simulink model "static_split_junction_test"  (R2014b)
settings: Solver=ode45  StartTime=0.0  StopTime=10.0  RelTol=1e-3
libraries: DAEMOT_Lib x7
settings Model: Creator=pangbor2  LastModifiedBy=pangbor2

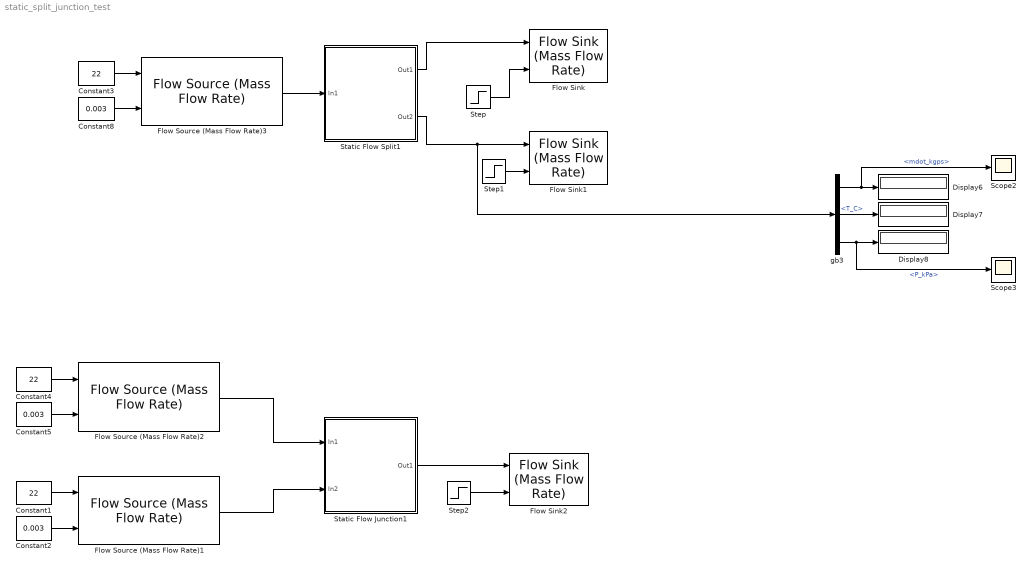
== system static_split_junction_test ==
  Constant1 : Constant  Value=22
  Constant2 : Constant  Value=0.003
  Constant3 : Constant  Value=22
  Constant4 : Constant  Value=22
  Constant5 : Constant  Value=0.003
  Constant8 : Constant  Value=0.003
  Display6 : Display
  Display7 : Display
  Display8 : Display
  Flow Sink : DAEMOT_Lib/Components/Flow Sink (Mass Flow Rate)  M_ext=on  M=0  T_ext=on  T=0  P_ext=on  P=0
  Flow Sink1 : DAEMOT_Lib/Components/Flow Sink (Mass Flow Rate)  M_ext=on  M=0  T_ext=on  T=0  P_ext=on  P=0
  Flow Sink2 : DAEMOT_Lib/Components/Flow Sink (Mass Flow Rate)  M_ext=on  M=0  T_ext=on  T=0  P_ext=on  P=0
  Flow Source (Mass Flow Rate)1 : DAEMOT_Lib/Components/Flow Source (Mass Flow Rate)  M_ext=on  M=0  T_ext=on  T=0  P_ext=on  P=0
  Flow Source (Mass Flow Rate)2 : DAEMOT_Lib/Components/Flow Source (Mass Flow Rate)  M_ext=on  M=0  T_ext=on  T=0  P_ext=on  P=0
  Flow Source (Mass Flow Rate)3 : DAEMOT_Lib/Components/Flow Source (Mass Flow Rate)  M_ext=on  M=0  T_ext=on  T=0  P_ext=on  P=0
  Scope2 : Scope
      settings: SaveName=ScopeData2
  Scope3 : Scope
      settings: SaveName=ScopeData3
  Static Flow Junction1 : Subsystem  AncestorBlock=DAEMOT_Lib/Components/Static Flow Junction  mask(Static Flow Junction){Num_In=2}
      mask prompts: Num_In "Number of Inlet Flows"
      mask help: Joins multiple flows into a single exit flow. Mass flow rates are taken from the upstream blocks. Note that the library link of the block is disabled when it is imported into a model.
      mask init:
      | h      = get_param(gcb,'handle');   % Get block handle
      | blk    = gcb; 
      | hblock = get(h);     % Parse out handles structure 
      | 
      | % delete any previous inports and bus selectors
      | for i = str2num(hblock.Num_In)+1:hblock.Ports(1)
      |     delete_block([blk,'/In',num2str(i)])
      |     delete_block([blk,'/b',num2str(i)])
      |     delete_block([blk,'/gm',num2str(i)])
      |     delete_block([blk,'/gt',num2str(i)])
      |     delete_block([blk,'/gp',num2str(i)])
      |     delete_block([blk,'/m',num2str(i)])
      |     delete_block([blk,'/p',num2str(i)])
      |     delete_block([blk,'/m2_',num2str(i)])
      |     delete_block([blk,'/t2_',num2str(i)])
      |     delete_block([blk,'/Divide',num2str(i)])
      |     
      | 	delete_unconnected_lines(blk)
      | end
      | 
      | % add the correct number of inputs to the add blocks
      | set_param([blk,'/Add'],'Inputs',char(repmat('+',1,str2num(hblock.Num_In))))
      | set_param([blk,'/Add1'],'Inputs',char(repmat('+',1,str2num(hblock.Num_In))))
      | set_param([blk,'/Add2'],'Inputs',char(repmat('+',1,str2num(hblock.Num_In))))
      | set_param([blk,'/Constant'],'Value',char(hblock.Num_In))
      | 
      | % generate inports, bus selectors, and route lines to each vector concat
      | for i = hblock.Ports(1)+1:str2num(hblock.Num_In)
      |     
      |     % add blocks
      |     add_block('simulink/Ports & Subsystems/In1',     [blk,'/In',num2str(i)],    'Position',[120 i*80-7 150 i*80+7]);         % adding inport   
      |     add_block([blk,'/b1'],                           [blk,'/b',num2str(i)],     'Position',[200 i*80-20+20-18 205 i*80-2+20+2]);         % adding inport
      |     add_block('simulink/Signal Routing/Goto',        [blk,'/gm',num2str(i)],    'Position',[260 i*80-17 340 i*80-3]);         % adding inport
      |     add_block('simulink/Signal Routing/Goto',        [blk,'/gt',num2str(i)],    'Position',[260 i*80+3 340 i*80+17]);         % adding inport
      |     add_block('simulink/Signal Routing/Goto',        [blk,'/gp',num2str(i)],    'Position',[260 i*80+6 340 i*80+20]);         % adding inport
      |     add_block('simulink/Signal Routing/From',        [blk,'/m',num2str(i)],     'Position',[410 i*80-20 490 i*80-2]);         % adding inport
      |     add_block('simulink/Signal Routing/From',        [blk,'/p',num2str(i)],     'Position',[1445 i*80-20 1525 i*80-2]);         % adding inport
      |     add_block('simulink/Signal Routing/From',        [blk,'/m2_',num2str(i)],   'Position',[730 i*80-20 810 i*80-2]);         % adding inport
      |     add_block('simulink/Signal Routing/From',        [blk,'/t2_',num2str(i)],   'Position',[730 i*80-20+24 810 i*80+24]);         % adding inport
      |     add_block([blk,'/Divide1'],                      [blk,'/Divide',num2str(i)],'Position',[825 i*80-20-7 841 i*80+27]);         % adding inport
      |     
      |     % set goto and from tags
      |     set_param([blk,'/gm',num2str(i)],'GotoTag',char(horzcat('m_in',num2str(i))))
      |     set_param([blk,'/gt',num2str(i)],'GotoTag',char(horzcat('T_in',num2str(i))))
      |     set_param([blk,'/gp',num2str(i)],'GotoTag',char(horzcat('P_in',num2str(i))))
      |     set_param([blk,'/m',num2str(i)],'GotoTag',char(horzcat('m_in',num2str(i))))
      |     set_param([blk,'/p',num2str(i)],'GotoTag',char(horzcat('P_in',num2str(i))))
      |     set_param([blk,'/m2_',num2str(i)],'GotoTag',char(horzcat('m_in',num2str(i))))
      |     set_param([blk,'/t2_',num2str(i)],'GotoTag',char(horzcat('T_in',num2str(i))))
      |    % set_param([blk,'/b',num2str(i)],'Outputs','3')
      |     
      |     % add lines
      |     add_line(blk,['In',num2str(i),'/1'], ['b',num2str(i),'/1'],'AutoRouting','on')
      |     add_line(blk,['b',num2str(i),'/1'],  ['gm',num2str(i),'/1'],'AutoRouting','on')
      |     add_line(blk,['b',num2str(i),'/2'],  ['gt',num2str(i),'/1'],'AutoRouting','on')
      |     add_line(blk,['b',num2str(i),'/3'],  ['gp',num2str(i),'/1'],'AutoRouting','on')
      |     add_line(blk,['m',num2str(i),'/1'],  ['Add/',num2str(i)],'AutoRouting','on')
      |     add_line(blk,['p',num2str(i),'/1'],  ['Add2/',num2str(i)],'AutoRouting','on')
      |     add_line(blk,['m2_',num2str(i),'/1'], ['Divide',num2str(i),'/1'],'AutoRouting','on')
      |     add_line(blk,['t2_',num2str(i),'/1'], ['Divide',num2str(i),'/2'],'AutoRouting','on')
      |     add_line(blk,['Divide',num2str(i),'/1'], ['Add1/',num2str(i)],'AutoRouting','on')
      |     
      |     % set goto and from background colors
      |     set_param([blk,'/gm',num2str(i)],'BackgroundColor','yellow') 
      |     set_param([blk,'/gt',num2str(i)],'BackgroundColor','yellow') 
      |     set_param([blk,'/gp',num2str(i)],'BackgroundColor','yellow') 
      |     set_param([blk,'/m',num2str(i)],'BackgroundColor','cyan') 
      |     set_param([blk,'/p',num2str(i)],'BackgroundColor','cyan') 
      |     set_param([blk,'/m2_',num2str(i)],'BackgroundColor','cyan') 
      |     set_param([blk,'/t2_',num2str(i)],'BackgroundColor','cyan') 
      |         
      | end
      settings: CopyFcn=|
      | h      = get_param(gcb,'handle');   % Get block handle
      | blk    = gcb;
      | 
      | set_param(blk, 'LinkStatus', 'inactive')
      mask Display:
      | image(fliplr(imread('Split.jpg')));
      | 
      | text(0.5,0.95,['{\bf Static Flow Junction}'],'TexMode','on','horizontalAlignment', 'center')
      | 
      | port_label('output',1,['Flow Out'])
      | 
      | h      = get_param(gcb,'handle');   % Get block handle
      | blk    = gcb;
      | hblock = get(h);     % Parse out handles structure
      | for i = 1:str2num(hblock.Num_In)
      |     port_label('input',i,horzcat('Flow In #',num2str(i)))
      | end
  Static Flow Split1 : Subsystem  AncestorBlock=DAEMOT_Lib/Components/Static Flow Split  mask(Static Flow Split){Num_Out=2}
      mask prompts: Num_Out "Number of Outlet Flows"
      mask help: Splits an inlet flow into multiple exit flows. Mass flow rates are taken from the downstream blocks. Note that the library link of the block is disabled when it is imported into a model.
      mask init:
      | h      = get_param(gcb,'handle');   % Get block handle
      | blk    = gcb; 
      | hblock = get(h);     % Parse out handles structure 
      | 
      | % delete any previous inports and bus selectors
      | for i = str2num(hblock.Num_Out)+1:hblock.Ports(2)
      |    delete_block([blk,'/Out',num2str(i)])
      |    delete_block([blk,'/m',num2str(i)])
      |    delete_block([blk,'/t',num2str(i)])
      |    delete_block([blk,'/p',num2str(i)])
      |    delete_block([blk,'/b',num2str(i)])
      |    delete_block([blk,'/Source',num2str(i)])
      |    delete_block([blk,'/g',num2str(i)])
      |    
      |    delete_unconnected_lines(blk)
      | end
      | 
      | % add the correct number of inputs to the add block
      | set_param([blk,'/Add'],'Inputs',char(repmat('+',1,str2num(hblock.Num_Out))))
      | 
      | % generate inports, bus selectors, and route lines to each vector concat
      | for i = hblock.Ports(2)+1:str2num(hblock.Num_Out)
      |     
      |     % add blocks
      |     add_block('simulink/Ports & Subsystems/Out1',   [blk,'/Out',num2str(i)],   'Position',[30 i*80-25+20 60 i*80-12+20]);         % adding inport
      |     add_block('simulink/Signal Routing/From',       [blk,'/m',num2str(i)],     'Position',[-150 i*80-20 -70 i*80-2]);         % adding inport
      |     add_block('simulink/Signal Routing/From',       [blk,'/t',num2str(i)],     'Position',[-150 i*80-20+20 -70 i*80-2+20]);         % adding inport
      |     add_block('simulink/Signal Routing/From',       [blk,'/p',num2str(i)],     'Position',[-150 i*80-20+40 -70 i*80-2+40]);         % adding inport
      |     add_block('simulink/Signal Routing/Bus Creator',[blk,'/b',num2str(i)],     'Position',[5 i*80-20+20-18 10 i*80-2+20+2]);         % adding inport
      |     add_block('DAEMOT_Lib/Support Functions/Source',[blk,'/Source',num2str(i)],'Position',[395 i*80-14 460 i*80+14]);         % adding inport
      |     add_block('simulink/Signal Routing/Goto',       [blk,'/g',num2str(i)],     'Position',[505 i*80-9 585 i*80+9]);         % adding inport
      |     
      |     % set goto and from tags
      |     set_param([blk,'/m',num2str(i)],'GotoTag',char(horzcat('m_dot',num2str(i))))
      |     set_param([blk,'/t',num2str(i)],'GotoTag',char('T_in'))
      |     set_param([blk,'/p',num2str(i)],'GotoTag',char('P_in'))
      |     set_param([blk,'/g',num2str(i)],'GotoTag',char(['m_dot',num2str(i)]))
      |     set_param([blk,'/b',num2str(i)],'Inputs','3')
      |     
      |     % set goto and from background colors
      |     set_param([blk,'/t',num2str(i)],'BackgroundColor','cyan')
      |     set_param([blk,'/m',num2str(i)],'BackgroundColor','cyan') 
      |     set_param([blk,'/p',num2str(i)],'BackgroundColor','cyan') 
      |     set_param([blk,'/g',num2str(i)],'BackgroundColor','yellow')    
      |     
      |     % add lines
      |     add_line(blk,['m',num2str(i),'/1'],['b',num2str(i),'/1'],'AutoRouting','on')
      |     add_line(blk,['t',num2str(i),'/1'],['b',num2str(i),'/2'],'AutoRouting','on')
      |     add_line(blk,['p',num2str(i),'/1'],['b',num2str(i),'/3'],'AutoRouting','on')
      |     add_line(blk,['b',num2str(i),'/1'],['Out',num2str(i),'/1'],'AutoRouting','on')
      |     add_line(blk,['Source',num2str(i),'/1'],['g',num2str(i),'/1'],'AutoRouting','on')
      |     add_line(blk,['Source',num2str(i),'/1'],['Add/',num2str(i)],'AutoRouting','on')
      |     
      |     % set line names for mass flow bus
      |     p = get_param([blk,'/m',num2str(i)], 'PortHandles');
      |     l = get_param(p.Outport,'Line');
      |     set_param(l,'Name','mdot_kgps')
      |     
      |     % set line names for temperature bus
      |     p = get_param([blk,'/t',num2str(i)], 'PortHandles');
      |     l = get_param(p.Outport,'Line');
      |     set_param(l,'Name','T_C')
      |     
      |     % set line names for pressure bus
      |     p = get_param([blk,'/p',num2str(i)], 'PortHandles');
      |     l = get_param(p.Outport,'Line');
      |     set_param(l,'Name','P_kPa')
      | end
      | 
      | clear h blk hblock
      settings: CopyFcn=|
      | h      = get_param(gcb,'handle');   % Get block handle
      | blk    = gcb;
      | 
      | set_param(blk, 'LinkStatus', 'inactive')
      mask Display:
      | image(imread('Split.jpg'));
      | 
      | text(0.5,0.95,['{\bf Static Flow Split}'],'TexMode','on','horizontalAlignment', 'center')
      | 
      | port_label('input',1,['Flow In'])
      | 
      | h      = get_param(gcb,'handle');   % Get block handle
      | blk    = gcb;
      | hblock = get(h);     % Parse out handles structure
      | for i = 1:str2num(hblock.Num_Out)
      |     port_label('output',i,horzcat('Flow Out #',num2str(i)))
      | end
  Step : Step  Time=100  Before=.002  After=.003  SampleTime=0
  Step1 : Step  Time=100  Before=.002  After=.003  SampleTime=0
  Step2 : Step  Time=100  Before=.002  After=.003  SampleTime=0
  gb3 : BusSelector  OutputSignals=mdot_kgps,T_C,P_kPa
  wires:
  Flow Source (Mass Flow Rate)3/1 -> Static Flow Split1/1(In1)
  Step/1 -> Flow Sink/2
  Static Flow Split1/1(Out1) -> Flow Sink/1
  Step1/1 -> Flow Sink1/2
  Step2/1 -> Flow Sink2/2
  Static Flow Junction1/1(Out1) -> Flow Sink2/1
  gb3/2 -> Display7/1  "<T_C>"
  gb3/1 -> Scope2/1, Display6/1  "<mdot_kgps>"
  Static Flow Split1/2(Out2) -> gb3/1, Flow Sink1/1
  gb3/3 -> Scope3/1, Display8/1  "<P_kPa>"
  Constant8/1 -> Flow Source (Mass Flow Rate)3/2
  Constant3/1 -> Flow Source (Mass Flow Rate)3/1
  Constant5/1 -> Flow Source (Mass Flow Rate)2/2
  Constant4/1 -> Flow Source (Mass Flow Rate)2/1
  Constant2/1 -> Flow Source (Mass Flow Rate)1/2
  Constant1/1 -> Flow Source (Mass Flow Rate)1/1
  Flow Source (Mass Flow Rate)2/1 -> Static Flow Junction1/1(In1)
  Flow Source (Mass Flow Rate)1/1 -> Static Flow Junction1/2(In2)

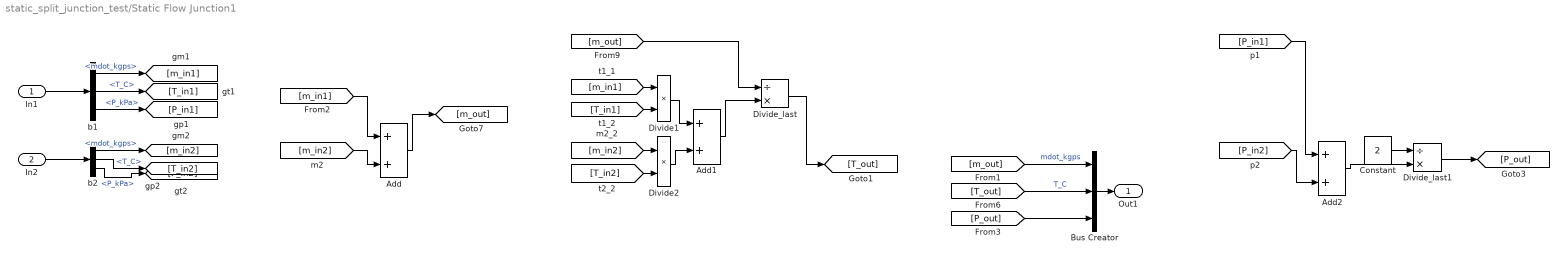
== system static_split_junction_test/Static Flow Junction1 ==
  In1 : Inport
  In2 : Inport  Port=2
  Add : Sum
  Add1 : Sum
  Add2 : Sum
  Bus Creator : BusCreator  Inputs=3
  Constant : Constant  Value=2
  Divide1 : Product  Inputs=**
  Divide2 : Product  Inputs=**
  Divide_last : Product  Inputs=/*
  Divide_last1 : Product  Inputs=/*
  b1 : BusSelector  OutputSignals=mdot_kgps,T_C,P_kPa
  b2 : BusSelector  OutputSignals=mdot_kgps,T_C,P_kPa
  Out1 : Outport
  wires:
  Divide1/1 -> Add1/1
  Add1/1 -> Divide_last/2
  [T_in1] -> Divide1/2
  [m_in1] -> Divide1/1
  Divide_last/1 -> [T_out]
  [m_in1] -> Add/1
  Add/1 -> [m_out]
  [T_out] -> Bus Creator/2  "T_C"
  [m_out] -> Bus Creator/1  "mdot_kgps"
  Bus Creator/1 -> Out1/1
  [m_out] -> Divide_last/1
  [P_out] -> Bus Creator/3
  b1/1 -> [m_in1]  "<mdot_kgps>"
  b1/2 -> [T_in1]  "<T_C>"
  In1/1 -> b1/1
  b1/3 -> [P_in1]  "<P_kPa>"
  [P_in1] -> Add2/1
  Add2/1 -> Divide_last1/2
  Divide_last1/1 -> [P_out]
  Constant/1 -> Divide_last1/1
  In2/1 -> b2/1
  b2/1 -> [m_in2]  "<mdot_kgps>"
  b2/2 -> [T_in2]  "<T_C>"
  b2/3 -> [P_in2]  "<P_kPa>"
  [m_in2] -> Add/2
  [P_in2] -> Add2/2
  [m_in2] -> Divide2/1
  [T_in2] -> Divide2/2
  Divide2/1 -> Add1/2

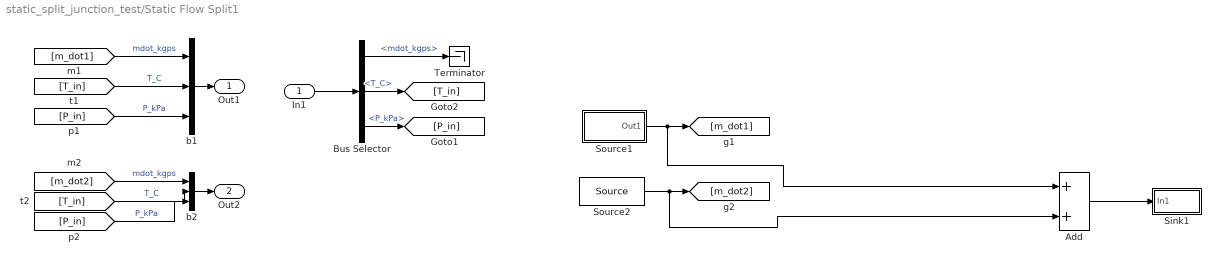
== system static_split_junction_test/Static Flow Split1 ==
  In1 : Inport
  Add : Sum
  Bus Selector : BusSelector  OutputSignals=mdot_kgps,T_C,P_kPa
  Sink1 : Subsystem
      settings: CopyFcn=rev_comms_sink()  NameChangeFcn=rev_comms_sink()
      mask Display: text(0.25,0.5,'Sink')
  Source1 : Subsystem
      mask init:
      | n_src = gcb;
      | n_src = str2num(n_src(end));
      | 
      | rev_comms_source(n_src);
      mask Display: text(0.25,0.5,'Source')
  Source2 : DAEMOT_Lib/Support Functions/Source
  Terminator : Terminator
  b1 : BusCreator  Inputs=3
  b2 : BusCreator  Inputs=3
  Out1 : Outport
  Out2 : Outport  Port=2
  wires:
  b1/1 -> Out1/1
  [m_dot1] -> b1/1  "mdot_kgps"
  Bus Selector/2 -> [T_in]  "<T_C>"
  [T_in] -> b1/2  "T_C"
  Bus Selector/1 -> Terminator/1  "<mdot_kgps>"
  Source1/1(Out1) -> [m_dot1], Add/1
  In1/1 -> Bus Selector/1
  Add/1 -> Sink1/1(In1)
  [P_in] -> b1/3  "P_kPa"
  Bus Selector/3 -> [P_in]  "<P_kPa>"
  [m_dot2] -> b2/1  "mdot_kgps"
  [T_in] -> b2/2  "T_C"
  [P_in] -> b2/3  "P_kPa"
  b2/1 -> Out2/1
  Source2/1 -> [m_dot2], Add/2

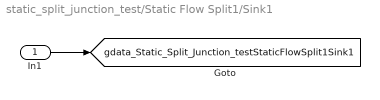
== system static_split_junction_test/Static Flow Split1/Sink1 ==
  In1 : Inport
  tag scope: gdata_Static_Split_Junction_testStaticFlowSplit1Sink1=global
  wires:
  In1/1 -> [gdata_Static_Split_Junction_testStaticFlowSplit1Sink1]

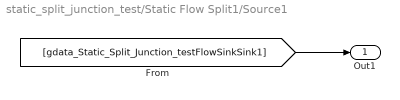
== system static_split_junction_test/Static Flow Split1/Source1 ==
  Out1 : Outport
  wires:
  [gdata_Static_Split_Junction_testFlowSinkSink1] -> Out1/1
